simulink model "plant_model"  (R2023b)
settings: Solver=VariableStepAuto  StartTime=0.0  StopTime=10.0  RelTol=1e-3
undefined symbols (not defined in the file): sysc, x0
libraries: fl_lib x10, nesl_utility x4
(part 1 of 3)
settings Model: Creator=MPC5  LastModifiedBy=block

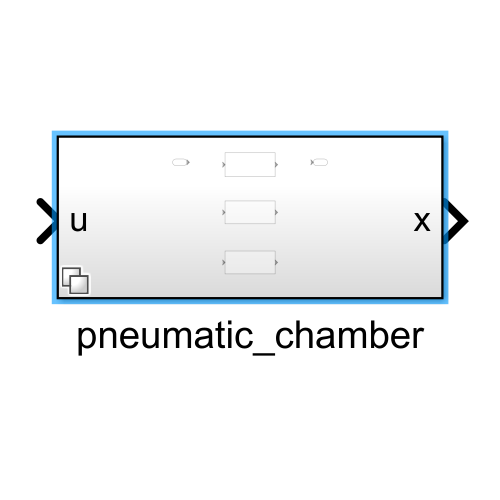
[thumbnail: Simulink's stored preview of the top-level diagram]
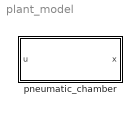
== system plant_model ==
  pneumatic_chamber : Subsystem  Variant=on

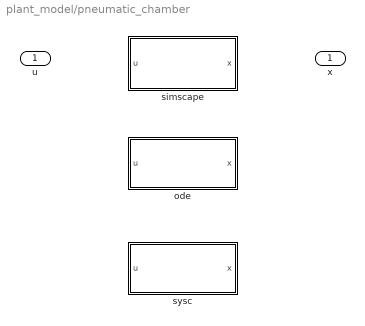
== system plant_model/pneumatic_chamber ==
  u : Inport
  ode : Subsystem  VariantControl="plant_model_type==\"ode\""
  simscape : Subsystem  VariantControl="plant_model_type==\"simscape\""
  sysc : Subsystem  VariantControl="plant_model_type==\"sysc\""
  x : Outport

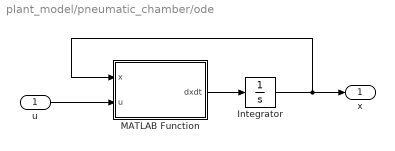
== system plant_model/pneumatic_chamber/ode ==
  u : Inport
  Integrator : Integrator  InitialCondition=x0
  MATLAB Function : MATLAB Function  TreatAsAtomicUnit=on
  x : Outport
  wires:
  MATLAB Function/1(dxdt) -> Integrator/1
  u/1 -> MATLAB Function/2(u)
  Integrator/1 -> x/1, MATLAB Function/1(x)
